simulink model "BalanceCar"  (R2022a)
settings: Solver=FixedStepDiscrete  StartTime=0.0  StopTime=inf  FixedStep=0.001  MaxStep=1e-3  RelTol=1e-3
values from neighbouring files (symbols this model uses):
  BALANCE_KD = 0.09    [BalanceCar.sldd]
  BALANCE_KP = 40.0    [BalanceCar.sldd]
  DIRECTION_KD = 0.1    [BalanceCar.sldd]
  DIRECTION_KP = 10.0    [BalanceCar.sldd]
  HIGH = 1.0    [BalanceCar.sldd]
  LOW = 0.0    [BalanceCar.sldd]
  MAX_PWM = 999.0    [BalanceCar.sldd]
  MIN_PWM = 900.0    [BalanceCar.sldd]
  NUM0 = 0.0    [BalanceCar.sldd]
  SPEED_KD = 0.0    [BalanceCar.sldd]
  SPEED_KI = 0.01    [BalanceCar.sldd]
  SPEED_KP = 18.0    [BalanceCar.sldd]
libraries: slpidlib x1
settings Model: DataDictionary=BalanceCar.sldd  Creator=Jepson  LastModifiedBy=Jepson
settings OptimizationCC: StrengthReduction=on  PassReuseOutputArgsAs=Individual arguments  ZeroExternalMemoryAtStartup=off  ZeroInternalMemoryAtStartup=off  NoFixptDivByZeroProtection=on  EfficientFloat2IntCast=on  OptimizeBlockOrder=speed  OptimizationPriority=Speed  MultiThreadedLoops=on  EfficientTunableParamExpr=on
settings DebuggingCC: ParameterPrecisionLossMsg=none  ParameterTunabilityLossMsg=error
settings HardwareCC: ProdBitPerPointer=32  ProdBitPerSizeT=32  ProdBitPerPtrDiffT=32  ProdLargestAtomicFloat=None  ProdWordSize=32  ProdHWDeviceType=Custom Processor->Custom Processor  TargetIntDivRoundTo=Zero  TargetEndianess=LittleEndian  TargetHWDeviceType=Custom Processor->Custom Processor  ProdEqTarget=off
settings ModelReferenceCC: ModelReferenceNumInstancesAllowed=Single
settings SFSimCC: MATLABDynamicMemAlloc=off
settings RTWCC: SystemTargetFile=ert.tlc  GenCodeOnly=on  TemplateMakefile=ert_default_tmf
settings CodeAppCC: ForceParamTrailComments=on  IgnoreCustomStorageClasses=off  OperatorAnnotations=on  SimulinkDataObjDesc=on  SFDataObjDesc=on  InsertBlockDesc=on
settings ERTTargetCC: TargetLangStandard=C99 (ISO)  GenerateSampleERTMain=on  IncludeMdlTerminateFcn=off  SupportNonFinite=off  SupportComplex=off  RemoveDisableFunc=on  ERTCustomFileTemplate=example_file_process.tlc  ERTFilePackagingFormat=CompactWithDataFile

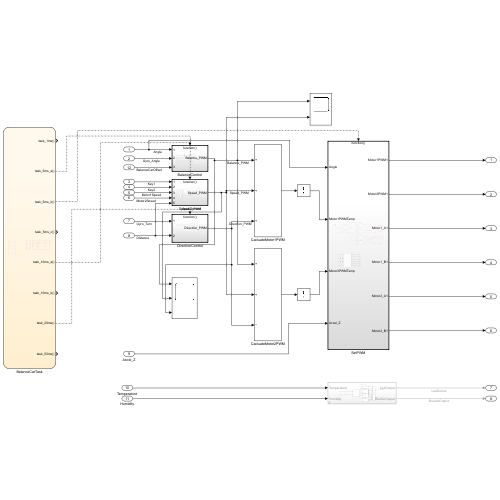
[thumbnail: Simulink's stored preview of the top-level diagram]
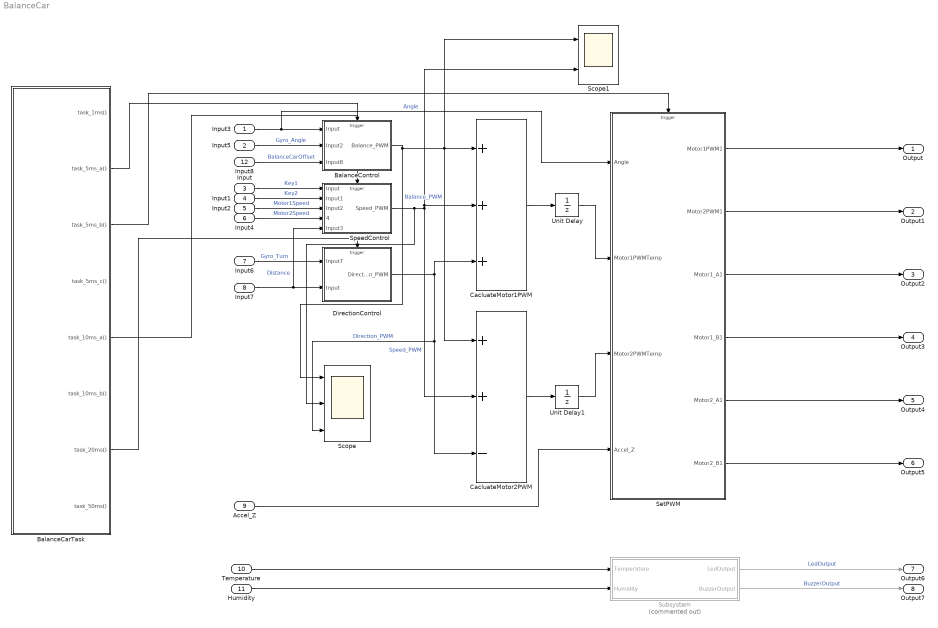
== system BalanceCar ==
  Input3 : Inport
  Input5 : Inport  Port=2
  Input : Inport  Port=3
  Input1 : Inport  Port=4
  Input2 : Inport  Port=5
  Input4 : Inport  Port=6
  Input6 : Inport  Port=7
  Input7 : Inport  Port=8
  Accel_Z : Inport  Port=9
  Temperature : Inport  Port=10
  Humidity : Inport  Port=11
  Input8 : Inport  Port=12
  BalanceCarTask : Stateflow chart  TreatAsAtomicUnit=on
      settings: PortSchema="{\"entries\":[{\"content\":{\"sides\":[{\"content\":{\"connectorIds\":[]},\"type\":\"ConnectorPlacement.EquallySpacedRectSide\",\"uuid\":\"98753e40-222e-4eaa-8b46-951d80aed91d\"},{\"content\":{\"connectorIds\":[\"Out2\",\"Out3\",\"Out5\",\"Out6\",\"Out1\",\"Out7\",\"Out4\",\"Out8\"],\"side\":\"RIGHT\"},\"type\":\"ConnectorPlacement.EquallySpacedRectSide\",\"uuid\":\"89dfa4e3-f29a-46ce-86e2-d4de18f5cc28\"},{\"content\":{\"connectorIds\":[],\"side\":\"TOP\"},\"type\":\"ConnectorPlacement.EquallySpacedRectSide\",\"uuid\":\"b5891d09-d472-4237-aaa4-93c027884cfd\"}]},\"type\":\"ConnectorPlacement.EquallySpacedConnector\",\"uuid\":\"b61f173b-e366-4c49-aaca-29ddc1ea1eb2\"}],\"packageUris\":[\"http://schema.mathworks.com/mf0/Connector/R2020b\"],\"version\":\"1.0\"}"
  BalanceControl : Subsystem  TreatAsAtomicUnit=on
      settings: RTWFcnNameOpts=Use subsystem name
  CacluateMotor1PWM : Sum  Inputs=+++
  CacluateMotor2PWM : Sum  Inputs=++-
  DirectionControl : Subsystem  TreatAsAtomicUnit=on  RTWFcnName=DirectionControl
      settings: RTWSystemCode=Nonreusable function  RTWFcnNameOpts=User specified
  Scope : Scope  NumInputPorts=3
  Scope1 : Scope  NumInputPorts=2
  SetPWM : Subsystem  TreatAsAtomicUnit=on
      settings: RTWFcnNameOpts=Use subsystem name
  SpeedControl : Subsystem  TreatAsAtomicUnit=on  RTWFcnName=SpeedControl
      settings: RTWSystemCode=Nonreusable function  RTWFcnNameOpts=User specified
  Subsystem : Subsystem  Commented=on
  Unit Delay : UnitDelay  SampleTime=-1  HasFrameUpgradeWarning=on
  Unit Delay1 : UnitDelay  SampleTime=-1  HasFrameUpgradeWarning=on
  Output : Outport
  Output1 : Outport  Port=2
  Output2 : Outport  Port=3
  Output3 : Outport  Port=4
  Output4 : Outport  Port=5
  Output5 : Outport  Port=6
  Output6 : Outport  Port=7
  Output7 : Outport  Port=8
  wires:
  Input/1 -> SpeedControl/1(Input)  "Key1"
  Input1/1 -> SpeedControl/2(Input1)  "Key2"
  Input2/1 -> SpeedControl/3(Input2)  "Motor1Speed"
  BalanceCarTask/3(task_5ms_a()) -> BalanceControl/Trigger
  Input3/1 -> BalanceControl/1(Input), SetPWM/1(Angle)  "Angle"
  Input5/1 -> BalanceControl/2(Input2)  "Gyro_Angle"
  BalanceControl/1(Balance_PWM) -> Scope1/1, CacluateMotor2PWM/1, CacluateMotor1PWM/1, Scope/1  "Balance_PWM"
  SpeedControl/1(Speed_PWM) -> Scope/2, Scope1/2, CacluateMotor1PWM/2, CacluateMotor2PWM/2  "Speed_PWM"
  SetPWM/1(Motor1PWM1) -> Output/1
  SetPWM/2(Motor2PWM1) -> Output1/1
  SetPWM/3(Motor1_A1) -> Output2/1
  SetPWM/4(Motor1_B1) -> Output3/1
  SetPWM/5(Motor2_A1) -> Output4/1
  SetPWM/6(Motor2_B1) -> Output5/1
  CacluateMotor1PWM/1 -> Unit Delay/1
  CacluateMotor2PWM/1 -> Unit Delay1/1
  Unit Delay/1 -> SetPWM/2(Motor1PWMTemp)
  Unit Delay1/1 -> SetPWM/3(Motor2PWMTemp)
  Input4/1 -> SpeedControl/4(4)  "Motor2Speed"
  BalanceCarTask/5(task_5ms_b()) -> SetPWM/Trigger
  BalanceCarTask/1(task_10ms_a()) -> SpeedControl/Trigger
  BalanceCarTask/4(task_20ms()) -> DirectionControl/Trigger
  Input7/1 -> SpeedControl/5(Input3), DirectionControl/2(Input)  "Distance"
  Input6/1 -> DirectionControl/1(Input7)  "Gyro_Turn"
  DirectionControl/1(Direction_PWM) -> CacluateMotor1PWM/3, CacluateMotor2PWM/3, Scope/3  "Direction_PWM"
  Accel_Z/1 -> SetPWM/4(Accel_Z)
  Temperature/1 -> Subsystem/1(Temperature)
  Humidity/1 -> Subsystem/2(Humidity)
  Subsystem/1(LedOutput) -> Output6/1  "LedOutput"
  Subsystem/2(BuzzerOutput) -> Output7/1  "BuzzerOutput"
  Input8/1 -> BalanceControl/3(Input8)  "BalanceCarOffset"

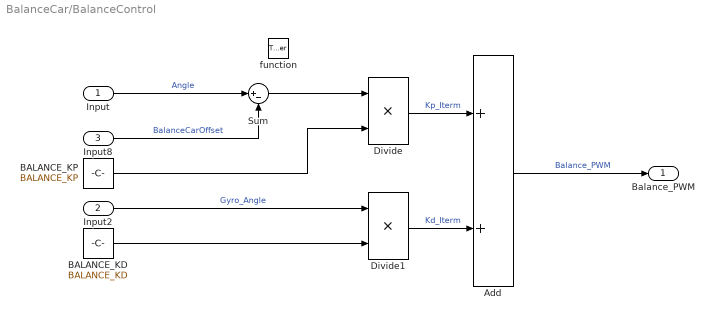
== system BalanceCar/BalanceControl ==
  Input : Inport
  Input2 : Inport  Port=2
  Input8 : Inport  Port=3
  function : TriggerPort  TriggerType=function-call  VariantControl=(inherit)
  Add : Sum  OutDataTypeStr=int16
  BALANCE_KD : Constant  Value=BALANCE_KD
  BALANCE_KP : Constant  Value=BALANCE_KP
  Divide : Product  Inputs=**
  Divide1 : Product  Inputs=**
  Sum : Sum  Inputs=|+-
  Balance_PWM : Outport
  wires:
  Input/1 -> Sum/1  "Angle"
  Sum/1 -> Divide/1
  Divide/1 -> Add/1  "Kp_Iterm"
  Input2/1 -> Divide1/1  "Gyro_Angle"
  Divide1/1 -> Add/2  "Kd_Iterm"
  Add/1 -> Balance_PWM/1  "Balance_PWM"
  Input8/1 -> Sum/2  "BalanceCarOffset"
  BALANCE_KP/1 -> Divide/2
  BALANCE_KD/1 -> Divide1/2

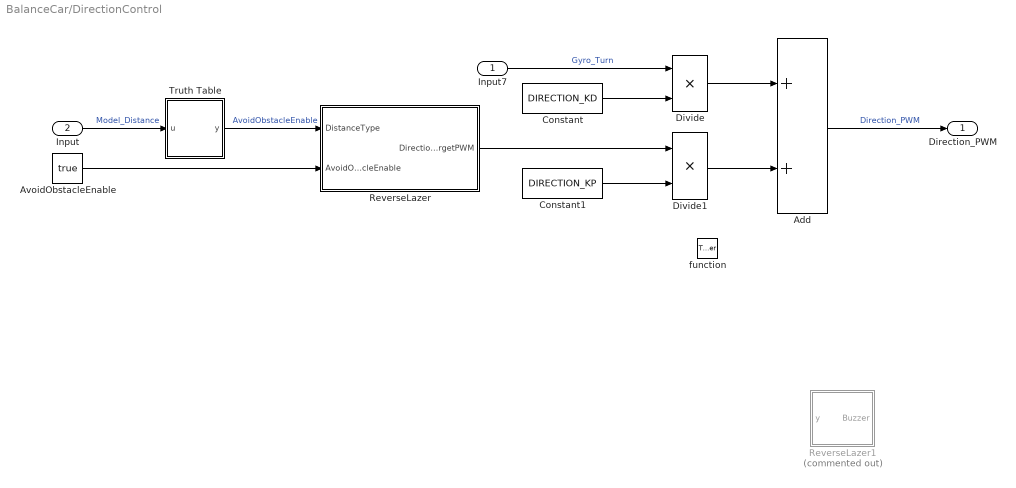
== system BalanceCar/DirectionControl ==
  Input7 : Inport
  Input : Inport  Port=2
  function : TriggerPort  TriggerType=function-call  VariantControl=(inherit)
  Add : Sum  OutDataTypeStr=int16
  AvoidObstacleEnable : Constant  Value=true  OutDataTypeStr=boolean
  Constant : Constant  Value=DIRECTION_KD
  Constant1 : Constant  Value=DIRECTION_KP
  Divide : Product  Inputs=**
  Divide1 : Product  Inputs=**
  ReverseLazer : Stateflow chart  TreatAsAtomicUnit=on
  ReverseLazer1 : Stateflow chart  Commented=on  TreatAsAtomicUnit=on
  Truth Table : Truth Table  TreatAsAtomicUnit=on
      settings: RTWSystemCode=Nonreusable function
  Direction_PWM : Outport
  wires:
  Input/1 -> Truth Table/1(u)  "Model_Distance"
  Truth Table/1(y) -> ReverseLazer/1(DistanceType)  "AvoidObstacleEnable"
  Input7/1 -> Divide/1  "Gyro_Turn"
  Constant/1 -> Divide/2
  Constant1/1 -> Divide1/2
  Divide/1 -> Add/1
  Divide1/1 -> Add/2
  Add/1 -> Direction_PWM/1  "Direction_PWM"
  ReverseLazer/1(DirectionTargetPWM) -> Divide1/1
  AvoidObstacleEnable/1 -> ReverseLazer/2(AvoidObstacleEnable)

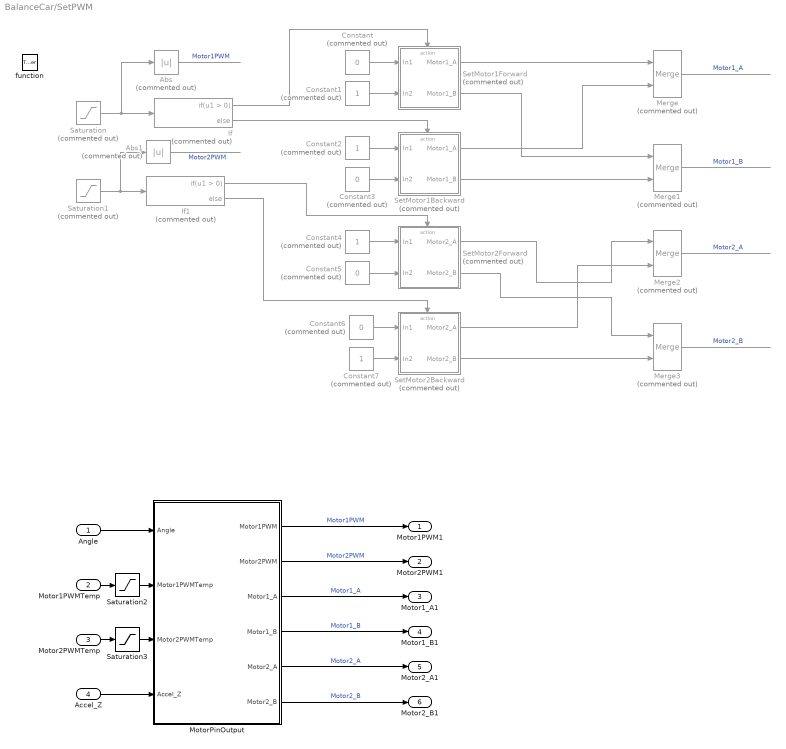
== system BalanceCar/SetPWM ==
  Angle : Inport
  Motor1PWMTemp : Inport  Port=2
  Motor2PWMTemp : Inport  Port=3
  Accel_Z : Inport  Port=4
  function : TriggerPort  TriggerType=function-call  VariantControl=(inherit)
  Abs : Abs  Commented=on  OutDataTypeStr=uint16  SaturateOnIntegerOverflow=off
  Abs1 : Abs  Commented=on  OutDataTypeStr=uint16  SaturateOnIntegerOverflow=off
  Constant{,3,5..6} (4 alike) : Constant  Commented=on  Value=0  OutDataTypeStr=uint8
  Constant{1..2,4,7} (4 alike) : Constant  Commented=on  OutDataTypeStr=uint8
  If : If  Commented=on
  If1 : If  Commented=on
  Merge{,1..3} (4 alike) : Merge  Commented=on
  MotorPinOutput : Stateflow chart  TreatAsAtomicUnit=on
      settings: PortSchema="{\"entries\":[{\"content\":{\"sides\":[{\"content\":{\"connectorIds\":[\"In3\",\"In1\",\"In2\",\"In4\"]},\"type\":\"ConnectorPlacement.EquallySpacedRectSide\",\"uuid\":\"f3e6de76-1fe1-4774-9311-d7aaff92af40\"},{\"content\":{\"connectorIds\":[\"Out1\",\"Out2\",\"Out3\",\"Out4\",\"Out5\",\"Out6\"],\"side\":\"RIGHT\"},\"type\":\"ConnectorPlacement.EquallySpacedRectSide\",\"uuid\":\"9ddd8262-d02c-4418-a44c-aa5250dd09ec\"},{\"content\":{\"connectorIds\":[],\"side\":\"TOP\"},\"type\":\"ConnectorPlacement.EquallySpacedRectSide\",\"uuid\":\"74ca197d-86c3-441f-a010-8590a39af9cb\"}]},\"type\":\"ConnectorPlacement.EquallySpacedConnector\",\"uuid\":\"3610e4e7-604b-4874-a455-67045648e8e5\"}],\"packageUris\":[\"http://schema.mathworks.com/mf0/Connector/R2020b\"],\"version\":\"1.0\"}"
  Saturation : Saturate  Commented=on  UpperLimit=900  LowerLimit=-900  OutDataTypeStr=int16
  Saturation1 : Saturate  Commented=on  UpperLimit=900  LowerLimit=-900  OutDataTypeStr=int16
  Saturation2 : Saturate  UpperLimit=990  LowerLimit=-900
  Saturation3 : Saturate  UpperLimit=999  LowerLimit=-999
  SetMotor1Backward : Subsystem  Commented=on  TreatAsAtomicUnit=on
  SetMotor1Forward : Subsystem  Commented=on  TreatAsAtomicUnit=on
  SetMotor2Backward : Subsystem  Commented=on  TreatAsAtomicUnit=on
  SetMotor2Forward : Subsystem  Commented=on  TreatAsAtomicUnit=on
  Motor1PWM1 : Outport
  Motor2PWM1 : Outport  Port=2
  Motor1_A1 : Outport  Port=3
  Motor1_B1 : Outport  Port=4
  Motor2_A1 : Outport  Port=5
  Motor2_B1 : Outport  Port=6
  wires:
  If/1 -> SetMotor1Forward/Action
  Constant/1 -> SetMotor1Forward/1(In1)
  Constant1/1 -> SetMotor1Forward/2(In2)
  If/2 -> SetMotor1Backward/Action
  Constant3/1 -> SetMotor1Backward/2(In2)
  Constant2/1 -> SetMotor1Backward/1(In1)
  Abs/1 -> ?  "Motor1PWM"
  Abs1/1 -> ?  "Motor2PWM"
  Constant6/1 -> SetMotor2Backward/1(In1)
  Constant7/1 -> SetMotor2Backward/2(In2)
  If1/2 -> SetMotor2Backward/Action
  Constant5/1 -> SetMotor2Forward/2(In2)
  Constant4/1 -> SetMotor2Forward/1(In1)
  If1/1 -> SetMotor2Forward/Action
  SetMotor1Forward/1(Motor1_A) -> Merge/1
  SetMotor1Backward/1(Motor1_A) -> Merge/2
  Merge/1 -> ?  "Motor1_A"
  SetMotor1Backward/2(Motor1_B) -> Merge1/2
  SetMotor1Forward/2(Motor1_B) -> Merge1/1
  SetMotor2Forward/1(Motor2_A) -> Merge2/1
  SetMotor2Backward/1(Motor2_A) -> Merge2/2
  SetMotor2Forward/2(Motor2_B) -> Merge3/1
  SetMotor2Backward/2(Motor2_B) -> Merge3/2
  Merge1/1 -> ?  "Motor1_B"
  Merge2/1 -> ?  "Motor2_A"
  Merge3/1 -> ?  "Motor2_B"
  MotorPinOutput/5(Motor2_A) -> Motor2_A1/1  "Motor2_A"
  MotorPinOutput/6(Motor2_B) -> Motor2_B1/1  "Motor2_B"
  MotorPinOutput/2(Motor2PWM) -> Motor2PWM1/1  "Motor2PWM"
  MotorPinOutput/1(Motor1PWM) -> Motor1PWM1/1  "Motor1PWM"
  MotorPinOutput/4(Motor1_B) -> Motor1_B1/1  "Motor1_B"
  MotorPinOutput/3(Motor1_A) -> Motor1_A1/1  "Motor1_A"
  Saturation1/1 -> Abs1/1, If1/1
  Saturation/1 -> Abs/1, If/1
  Angle/1 -> MotorPinOutput/3(Angle)
  Motor1PWMTemp/1 -> Saturation2/1
  Motor2PWMTemp/1 -> Saturation3/1
  Saturation2/1 -> MotorPinOutput/1(Motor1PWMTemp)
  Saturation3/1 -> MotorPinOutput/2(Motor2PWMTemp)
  Accel_Z/1 -> MotorPinOutput/4(Accel_Z)

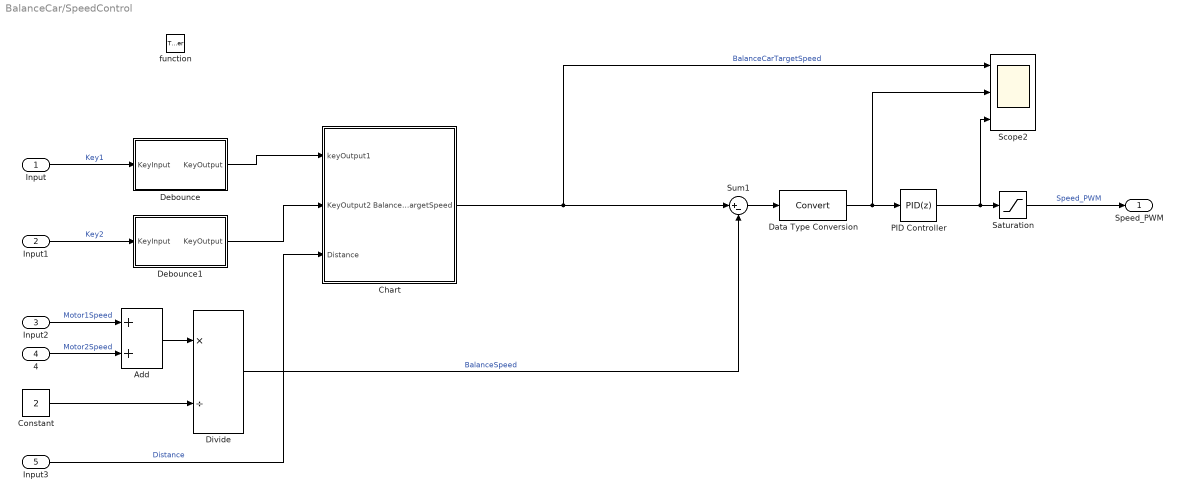
== system BalanceCar/SpeedControl ==
  Input : Inport
  Input1 : Inport  Port=2
  Input2 : Inport  Port=3
  4 : Inport  Port=4
  Input3 : Inport  Port=5
  function : TriggerPort  TriggerType=function-call  VariantControl=(inherit)
  Add : Sum
  Chart : Stateflow chart  TreatAsAtomicUnit=on
  Constant : Constant  Value=2  OutDataTypeStr=int8
  Data Type Conversion : DataTypeConversion  SaturateOnIntegerOverflow=off  RndMeth=Floor
  Debounce : Stateflow chart  TreatAsAtomicUnit=on
  Debounce1 : Stateflow chart  TreatAsAtomicUnit=on
  Divide : Product  Inputs=*/  OutDataTypeStr=int16
  PID Controller : slpidlib/PID Controller  Controller=PID  Form=Parallel  TimeDomain=Discrete-time  UseExternalTs=off  SampleTime=-1  IntegratorMethod=Forward Euler  FilterMethod=Forward Euler  ControllerParametersSource=internal  P=SPEED_KP  I=SPEED_KI  UseKiTs=on  D=SPEED_KD  N=100  UseFilter=on  TunerSelectOption=Transfer Function Based (PID Tuner App)  InitialConditionSource=internal  InitialConditionForIntegrator=0  InitialConditionForFilter=0  DifferentiatorICPrevScaledInput=0  ExternalReset=none  TrackingMode=off  Kt=1  LimitOutput=off  SatLimitsSource=internal  UpperSaturationLimit=MAX_PWM  LowerSaturationLimit=MIN_PWM  LinearizeAsGain=off  AntiWindupMode=none  Kb=1  POutMin=[]  POutMax=[]  IOutMin=[]  IOutMax=[]  DOutMin=[]  DOutMax=[]  NOutMin=[]  NOutMax=[]  SumOutDataTypeStr=int16  SumOutMin=[]  SumOutMax=[]  SaturationOutMin=[]  SaturationOutMax=[]  PParamMin=[]  PParamMax=[]  IParamMin=[]  IParamMax=[]  DParamMin=[]  DParamMax=[]  NParamMin=[]  NParamMax=[]  KbParamMin=[]  KbParamMax=[]  KtParamMin=[]  KtParamMax=[]  KbOutMin=[]  KbOutMax=[]  KtOutMin=[]  KtOutMax=[]  IntegratorOutMin=[]  IntegratorOutMax=[]  FilterOutMin=[]  FilterOutMax=[]  SumI1OutMin=[]  SumI1OutMax=[]  SumI2OutMin=[]  SumI2OutMax=[]  SumI3OutMin=[]  SumI3OutMax=[]  SumI4OutMin=[]  SumI4OutMax=[]  SumDOutMin=[]  SumDOutMax=[]  DifferentiatorOutMin=[]  DifferentiatorOutMax=[]  FilterDiffOutCoefMin=[]  FilterDiffOutCoefMax=[]  ReciprocalOutMin=[]  ReciprocalOutMax=[]  SumDenOutMin=[]  SumDenOutMax=[]  SumNumOutMin=[]  SumNumOutMax=[]  DivideOutMin=[]  DivideOutMax=[]  UdiffTsProdOutMin=[]  UdiffTsProdOutMax=[]  NTsProdOutMin=[]  NTsProdOutMax=[]  UintegralTsProdOutMin=[]  UintegralTsProdOutMax=[]  UngainTsProdOutMin=[]  UngainTsProdOutMax=[]  ClampingZeroOutDataTypeStr=Inherit: Inherit via back propagation  ClampingZeroOutMin=[]  ClampingZeroOutMax=[]  FilterDenConstantOutDataTypeStr=Inherit: Inherit via back propagation  FilterDenConstantOutMin=[]  FilterDenConstantOutMax=[]  PCopyOutDataTypeStr=Inherit: Inherit via back propagation  PCopyOutMin=[]  PCopyOutMax=[]  NCopyOutDataTypeStr=Inherit: Inherit via back propagation  NCopyOutMin=[]  NCopyOutMax=[]  IntegratorContinuousStateAttributes=''  IntegratorStateMustResolveToSignalObject=off  IntegratorRTWStateStorageClass=Auto  FilterContinuousStateAttributes=''  FilterStateMustResolveToSignalObject=off  FilterRTWStateStorageClass=Auto  ParallelPVariant=InternalParameters  IdealPVariant=Disabled  IVariant=InternalParameters  DVariant=InternalParameters  IntegratorVariant=Discrete  SatVariant=Disabled  AWVariant=Passthrough  PCopyVariant=Disabled  TRVariant=Disabled  FdbkBlocksVariant=Forward  IdealPFdbkVariant=Disabled  SatFdbkVariant=Disabled  DerivativeFilterVariant=ForwardEulerFilter  NVariant=InternalParameters  NCopyVariant=Disabled  FilterICVariant=InternalICsFilter  IntegratorICVariant=InternalICs  ExternalResetVariant=Disabled  TRSumVariant=Passthrough  SumFdbkVariant=Disabled  SumVariant=Sum_PID  TsampFilterVariant=InternalTs  TsampNgainVariant=Passthrough  TsampIntegralVariant=Passthrough  ExternalSaturationOutDataTypeStr=Inherit: Same as second input  aMode=0
  Saturation : Saturate  UpperLimit=900  LowerLimit=-900  OutDataTypeStr=int16
  Scope2 : Scope  NumInputPorts=3
  Sum1 : Sum  Inputs=|+-  InputSameDT=on  OutDataTypeStr=int16  LockScale=on
  Speed_PWM : Outport  OutDataTypeStr=int16
  wires:
  Input/1 -> Debounce/1(KeyInput)  "Key1"
  Debounce/1(KeyOutput) -> Chart/1(keyOutput1)
  Chart/1(BalanceCarTargetSpeed) -> Scope2/1, Sum1/1  "BalanceCarTargetSpeed"
  Debounce1/1(KeyOutput) -> Chart/2(KeyOutput2)
  Input1/1 -> Debounce1/1(KeyInput)  "Key2"
  Data Type Conversion/1 -> Scope2/2, PID Controller/1
  Sum1/1 -> Data Type Conversion/1
  PID Controller/1 -> Saturation/1, Scope2/3
  Input2/1 -> Add/1  "Motor1Speed"
  4/1 -> Add/2  "Motor2Speed"
  Add/1 -> Divide/1
  Constant/1 -> Divide/2
  Divide/1 -> Sum1/2  "BalanceSpeed"
  Saturation/1 -> Speed_PWM/1  "Speed_PWM"
  Input3/1 -> Chart/3(Distance)  "Distance"

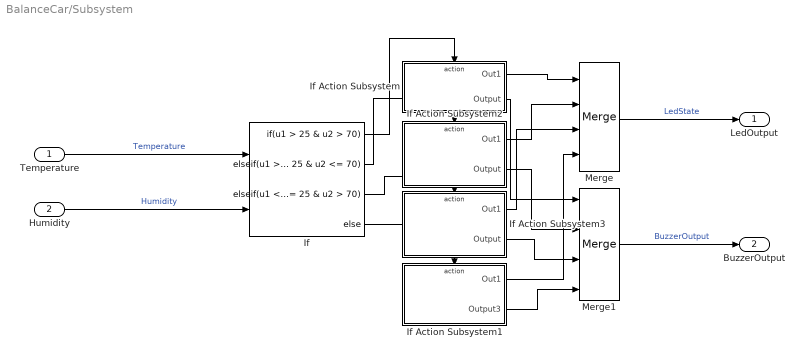
== system BalanceCar/Subsystem ==
  Temperature : Inport
  Humidity : Inport  Port=2
  If : If  NumInputs=2  IfExpression=u1 > 25 & u2 > 70  ElseIfExpressions=u1 > 25 & u2 <= 70,u1 <= 25 & u2 > 70
  If Action Subsystem : Subsystem  TreatAsAtomicUnit=on
  If Action Subsystem1 : Subsystem  TreatAsAtomicUnit=on
  If Action Subsystem2 : Subsystem  TreatAsAtomicUnit=on
  If Action Subsystem3 : Subsystem  TreatAsAtomicUnit=on
  Merge : Merge  Inputs=4
  Merge1 : Merge  Inputs=4
  LedOutput : Outport
  BuzzerOutput : Outport  Port=2
  wires:
  If/2 -> If Action Subsystem2/Action
  If/1 -> If Action Subsystem/Action
  If/4 -> If Action Subsystem1/Action
  If Action Subsystem1/2(Output3) -> Merge1/4
  If Action Subsystem3/2(Output) -> Merge1/3
  If Action Subsystem2/1(Out1) -> Merge/2
  If Action Subsystem2/2(Output) -> Merge1/2
  If Action Subsystem3/1(Out1) -> Merge/3
  If/3 -> If Action Subsystem3/Action
  If Action Subsystem1/1(Out1) -> Merge/4
  If Action Subsystem/2(Output) -> Merge1/1
  If Action Subsystem/1(Out1) -> Merge/1
  Temperature/1 -> If/1  "Temperature"
  Merge/1 -> LedOutput/1  "LedState"
  Merge1/1 -> BuzzerOutput/1  "BuzzerOutput"
  Humidity/1 -> If/2  "Humidity"

== system BalanceCar/SetPWM/MotorPinOutput/abs ==
  x : Inport  OutDataTypeStr=int16  PortDimensions=1
  f : TriggerPort  TriggerType=function-call  VariantControl=(inherit)
      settings: CopyFcn=Stateflow.SLINSF.SimulinkMan.removeBlockPreDeleteFcn  PreDeleteFcn=Stateflow.SLINSF.SimulinkMan.unsafePredeleteFcn
  Abs : Abs  OutDataTypeStr=uint16  SaturateOnIntegerOverflow=off
  y : Outport  OutDataTypeStr=uint16
  wires:
  x/1 -> Abs/1
  Abs/1 -> y/1

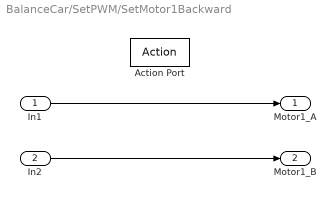
== system BalanceCar/SetPWM/SetMotor1Backward ==
  In1 : Inport
  In2 : Inport  Port=2
  Action Port : ActionPort  ActionPortLabel=else
  Motor1_A : Outport
  Motor1_B : Outport  Port=2
  wires:
  In2/1 -> Motor1_B/1
  In1/1 -> Motor1_A/1

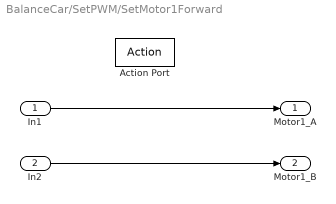
== system BalanceCar/SetPWM/SetMotor1Forward ==
  In1 : Inport
  In2 : Inport  Port=2
  Action Port : ActionPort  ActionPortLabel=if(u1 > 0)
  Motor1_A : Outport
  Motor1_B : Outport  Port=2
  wires:
  In2/1 -> Motor1_B/1
  In1/1 -> Motor1_A/1

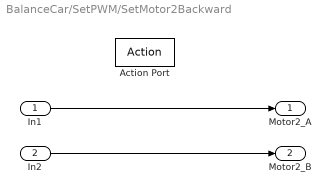
== system BalanceCar/SetPWM/SetMotor2Backward ==
  In1 : Inport
  In2 : Inport  Port=2
  Action Port : ActionPort  ActionPortLabel=else
  Motor2_A : Outport
  Motor2_B : Outport  Port=2
  wires:
  In1/1 -> Motor2_A/1
  In2/1 -> Motor2_B/1

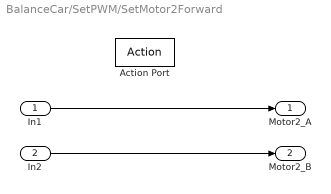
== system BalanceCar/SetPWM/SetMotor2Forward ==
  In1 : Inport
  In2 : Inport  Port=2
  Action Port : ActionPort  ActionPortLabel=if(u1 > 0)
  Motor2_A : Outport
  Motor2_B : Outport  Port=2
  wires:
  In1/1 -> Motor2_A/1
  In2/1 -> Motor2_B/1

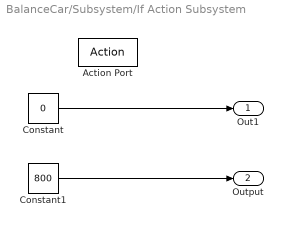
== system BalanceCar/Subsystem/If Action Subsystem ==
  Action Port : ActionPort  ActionPortLabel=if(u1 > 25 & u2 > 70)
  Constant : Constant  Value=0  OutDataTypeStr=uint8
  Constant1 : Constant  Value=800  OutDataTypeStr=uint16
  Out1 : Outport
  Output : Outport  Port=2
  wires:
  Constant/1 -> Out1/1
  Constant1/1 -> Output/1

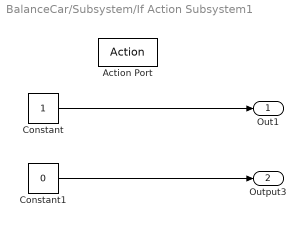
== system BalanceCar/Subsystem/If Action Subsystem1 ==
  Action Port : ActionPort  ActionPortLabel=else
  Constant : Constant  OutDataTypeStr=uint8
  Constant1 : Constant  Value=0  OutDataTypeStr=uint16
  Out1 : Outport
  Output3 : Outport  Port=2
  wires:
  Constant/1 -> Out1/1
  Constant1/1 -> Output3/1

== system BalanceCar/Subsystem/If Action Subsystem2 ==
  Action Port : ActionPort  ActionPortLabel=elseif(u1 > 25 & u2 <= 70)
  Constant : Constant  Value=0  OutDataTypeStr=uint8
  Constant1 : Constant  Value=0  OutDataTypeStr=uint16
  Out1 : Outport
  Output : Outport  Port=2
  wires:
  Constant1/1 -> Output/1
  Constant/1 -> Out1/1

== system BalanceCar/Subsystem/If Action Subsystem3 ==
  Action Port : ActionPort  ActionPortLabel=elseif(u1 <= 25 & u2 > 70)
  Constant : Constant  OutDataTypeStr=uint8
  Constant1 : Constant  Value=800  OutDataTypeStr=uint16
  Out1 : Outport
  Output : Outport  Port=2
  wires:
  Constant/1 -> Out1/1
  Constant1/1 -> Output/1

== stateflow chart BalanceCar/DirectionControl/ReverseLazer ==
  state Default [commented out]
    en:
    DirectionTargetPWM = 0;
    du:
    % disable chaoshengbo
    DiasbleAvoidObstacle = false;
  state TurnDirection [commented out]
    en:
    DirectionTargetPWM = 20;
    du:
    DirectionTargetPWM = DirectionTargetPWM - 1;
  state Back [commented out]
    en:
    DirectionTargetPWM = -20;
    du:
    DirectionTargetPWM = DirectionTargetPWM + 1;
  state Default1
    en:
    DirectionTargetPWM = 0;
  state TurnDirection1
    en:
    DirectionTargetPWM = 0;
    state Enter1
      du:
      DirectionTargetPWM = DirectionTargetPWM + 5;
    state End1
    (default) -> TurnDirection1.Enter1
    TurnDirection1.Enter1 -> TurnDirection1.End1 : [ DistanceType == 0 || DirectionTargetPWM > 100]
  state StopTurn
    en:
    state Enter1
      du:
      DirectionTargetPWM = DirectionTargetPWM - 10;
    state End1
    (default) -> StopTurn.Enter1
    StopTurn.Enter1 -> StopTurn.End1 : [DirectionTargetPWM == 0]
  state Back2 [commented out]
    en:
    DirectionTargetPWM = 40;
    state Enter1 [commented out]
      du:
      DirectionTargetPWM = DirectionTargetPWM - 4;
    state End1 [commented out]
    (default) -> Back2.Enter1 [commented out]
    Back2.Enter1 -> Back2.End1 [commented out] : [DirectionTargetPWM == 0]
  state Back1 [commented out]
    en:
    DirectionTargetPWM = 40;
    state Enter1 [commented out]
      du:
      DirectionTargetPWM = DirectionTargetPWM - 4;
    state End1 [commented out]
    (default) -> Back1.Enter1 [commented out]
    Back1.Enter1 -> Back1.End1 [commented out] : [DirectionTargetPWM == 0]
  (default) -> Default [commented out]
  Default -> TurnDirection [commented out] : [DiasbleAvoidObstacle...
      | &&(DistanceType == 1 || DistanceType == 2 || DistanceType == 3)]
  TurnDirection -> Back [commented out] : [(DirectionTargetPWM == 0)&&after(1000,msec)]
  Back -> Default [commented out] : [(DirectionTargetPWM == 0)&&after(1000,msec)]
  (default) -> Default1
  Default1 -> TurnDirection1 : [AvoidObstacleEnable...
      |  &&(DistanceType == 1)...
      |  &&(DistanceType == 2)...
      |  &&(DistanceType == 3)]
  TurnDirection1.End1 -> StopTurn : [after(10,msec)]
  StopTurn -> Default1 : [DirectionTargetPWM == 0 || DistanceType == 0]
  StopTurn.End1 -> Back2 [commented out] : [after(20,msec)]
  Back2.End1 -> Back1 [commented out] : [after(20,msec)]
  data: DirectionTargetPWM output; DistanceType input; AvoidObstacleEnable input

== matlab function BalanceCar/DirectionControl/Truth Table ==
  data: u input; y output uint8 =0
function y = fcn(u)

aVarTruthTableCondition_1 = false;
aVarTruthTableCondition_2 = false;
aVarTruthTableCondition_3 = false;


% Example condition 1

aVarTruthTableCondition_1 = logical((u  <= 10) &&(u  >=0));

% Example condition 2

aVarTruthTableCondition_2 = logical((u  <= 30) &&(u  > 10));

% Example condition 3

aVarTruthTableCondition_3 = logical((u  >30) &&(u  < 50));

if (aVarTruthTableCondition_1)
    aFcnTruthTableAction_1();
elseif (~aVarTruthTableCondition_1 && aVarTruthTableCondition_2)
    aFcnTruthTableAction_2();
elseif (~aVarTruthTableCondition_1 && ~aVarTruthTableCondition_2 && aVarTruthTableCondition_3)
    aFcnTruthTableAction_3();
else % Default
    aFcnTruthTableAction_4();
end

function aFcnTruthTableAction_1()

% Action 1:Dangerous

y = 1;

function aFcnTruthTableAction_2()

% Action 2: Carefull

y = 2;

function aFcnTruthTableAction_3()

% Action 3:Warning

y = 3;

function aFcnTruthTableAction_4()

% Action 4:Noramal

y = 0;

== stateflow chart BalanceCar/BalanceCarTask ==
  state Task_5ms [function]
    (default) -> (junction 132)
    (junction 132) -> (junction 140) [order 1] : [task_5ms_count == 1]
    (junction 132) -> (junction 144) [order 2]
    (junction 140) -> (junction 142) : {task_5ms_a}
    (junction 142) -> (junction 144)
    (junction 144) -> (junction 148)
    (junction 148) -> (junction 155) [order 1] : [task_5ms_count == 2]
    (junction 148) -> (junction 151) [order 2]
    (junction 155) -> (junction 152) : {task_5ms_b}
    (junction 152) -> (junction 151)
    (junction 151) -> (junction 162)
    (junction 162) -> (junction 166) [order 1] : [task_5ms_count == 3]
    (junction 162) -> (junction 160) [order 2]
    (junction 166) -> (junction 161) : {task_5ms_c}
    (junction 161) -> (junction 160)
  state Task_10ms [function]
    (default) -> (junction 169)
    (junction 169) -> (junction 193) [order 1] : [task_10ms_count == 2]
    (junction 169) -> (junction 181) [order 2]
    (junction 193) -> (junction 190) : {task_10ms_a}
    (junction 190) -> (junction 181)
    (junction 181) -> (junction 185)
    (junction 185) -> (junction 189) [order 1] : [task_10ms_count == 3]
    (junction 185) -> (junction 183) [order 2]
    (junction 189) -> (junction 184) : {task_10ms_b}
    (junction 184) -> (junction 183)
  state Task_20ms [function]
    (default) -> (junction 196)
    (junction 196) -> (junction 204) [order 1] : [task_20ms_count == 3]
    (junction 196) -> (junction 201) [order 2]
    (junction 204) -> (junction 202) : {task_20ms}
    (junction 202) -> (junction 201)
  state Task_50ms [function]
    (default) -> (junction 206)
    (junction 206) -> (junction 214) [order 1] : [task_50ms_count == 4]
    (junction 206) -> (junction 211) [order 2]
    (junction 214) -> (junction 212) : {task_50ms}
    (junction 212) -> (junction 211)
  (default) -> (junction 87) : {task_5ms_count = task_5ms_count + 1;}
  (junction 87) -> (junction 69) : {task_1ms;}
  (junction 69) -> (junction 77) [order 1] : [mod(task_5ms_count,5)==0]
  (junction 69) -> (junction 71) [order 2]
  (junction 77) -> (junction 79) : {task_5ms_count = 0;}
  (junction 79) -> (junction 71)
  (junction 71) -> (junction 93) : {task_10ms_count = task_10ms_count + 1;}
  (junction 93) -> (junction 95) [order 1] : [mod(task_10ms_count,10)==0]
  (junction 93) -> (junction 97) [order 2]
  (junction 95) -> (junction 99) : {task_10ms_count = 0;}
  (junction 99) -> (junction 97)
  (junction 97) -> (junction 106) : {task_20ms_count = task_20ms_count + 1;}
  (junction 106) -> (junction 108) [order 1] : [mod(task_20ms_count,20)==0]
  (junction 106) -> (junction 103) [order 2]
  (junction 108) -> (junction 109) : {task_20ms_count = 1;}
  (junction 109) -> (junction 103)
  (junction 103) -> (junction 114) : {task_50ms_count = task_50ms_count + 1;}
  (junction 114) -> (junction 117) [order 1] : [mod(task_50ms_count,50)==0]
  (junction 114) -> (junction 115) [order 2]
  (junction 117) -> (junction 116) : {task_50ms_count = 0;}
  (junction 116) -> (junction 115)
  (junction 115) -> (junction 138) : {Task_5ms();
      | Task_10ms();
      | Task_20ms();
      | Task_50ms();}
  data: task_5ms_count local uint8 =NUM0; task_10ms_count local uint8 =NUM0; task_20ms_count local uint8 =NUM0; task_50ms_count local uint8 =NUM0
  events: task_10ms_a output FUNCTION_CALL_EVENT; task_1ms output FUNCTION_CALL_EVENT; task_5ms_a output FUNCTION_CALL_EVENT; task_20ms output FUNCTION_CALL_EVENT; task_5ms_b output FUNCTION_CALL_EVENT; task_5ms_c output FUNCTION_CALL_EVENT; task_10ms_b output FUNCTION_CALL_EVENT; task_50ms output FUNCTION_CALL_EVENT

== stateflow chart BalanceCar/SpeedControl/Debounce ==
  state Debounce [parallel]
    settings: executionOrder=1
    state Key1Off
      du:
      KeyState = OFF;
    state KeyOn
      du:
      KeyState = ON;
      KeyOnFlag = true;
    (default) -> Key1Off
    Key1Off -> KeyOn : [duration(KeyInput <= NUM0)>=0.01]
    KeyOn -> Key1Off : [duration(KeyInput > NUM0)>=0.01]
  state KeyCounter [function]
    (default) -> (junction 40)
    (junction 40) -> (junction 43) [order 1] : [(KeyOnFlag == true)&&(KeyState == OFF)]
    (junction 40) -> (junction 41) [order 2]
    (junction 43) -> (junction 37) : {KeyOnFlag = false;
        | KeyOutput =  ON;}
    (junction 41) -> (junction 37) : {KeyOutput =  OFF;}
  state KeyTimes [parallel]
    du:
    KeyCounter();
    settings: executionOrder=2
  data: KeyInput input uint8; OFF parameter; ON parameter; NUM0 parameter; KeyOutput output uint8; KeyOnFlag local boolean =false; KeyState local uint8 =OFF

== stateflow chart BalanceCar/SpeedControl/Debounce1 ==
  state Debounce [parallel]
    settings: executionOrder=1
    state Key1Off
      du:
      KeyState = OFF;
    state KeyOn
      du:
      KeyState = ON;
      KeyOnFlag = true;
    (default) -> Key1Off
    Key1Off -> KeyOn : [duration(KeyInput <= NUM0)>=0.01]
    KeyOn -> Key1Off : [duration(KeyInput > NUM0)>=0.01]
  state KeyCounter [function]
    (default) -> (junction 40)
    (junction 40) -> (junction 43) [order 1] : [(KeyOnFlag == true)&&(KeyState == OFF)]
    (junction 40) -> (junction 41) [order 2]
    (junction 43) -> (junction 37) : {KeyOnFlag = false;
        | KeyOutput =  ON;}
    (junction 41) -> (junction 37) : {KeyOutput =  OFF;}
  state KeyTimes [parallel]
    du:
    KeyCounter();
    settings: executionOrder=2
  data: KeyInput input uint8; OFF parameter; ON parameter; NUM0 parameter; KeyOutput output uint8; KeyOnFlag local boolean =false; KeyState local uint8 =OFF

== stateflow chart BalanceCar/SpeedControl/Chart ==
  state SpeedDown [function]
    (default) -> (junction 33)
    (junction 33) -> (junction 35) [order 1] : [KeyOutput2 == ON]
    (junction 33) -> (junction 37) [order 2]
    (junction 35) -> (junction 41) : {BalanceCarTargetSpeed=BalanceCarTargetSpeed-20;}
    (junction 37) -> (junction 41)
  state SpeedUp [function]
    (default) -> (junction 26)
    (junction 26) -> (junction 28) [order 1] : [keyOutput1 == ON]
    (junction 26) -> (junction 30) [order 2]
    (junction 28) -> (junction 23) : {BalanceCarTargetSpeed=BalanceCarTargetSpeed+20;}
    (junction 30) -> (junction 23)
  state SpeedUpStatus
    en:
    BalanceCarTargetSpeed = 0;
    du:
    SpeedUp();
    SpeedDown();
    SpeedStop();
  state SpeedStop [function]
    (default) -> (junction 58)
    (junction 58) -> (junction 59) [order 1] : [Distance <= 10]
    (junction 58) -> (junction 60) [order 2]
    (junction 59) -> (junction 61)
    (junction 60) -> (junction 61)
  (default) -> SpeedUpStatus
  data: keyOutput1 input; ON parameter; KeyOutput2 input; BalanceCarTargetSpeed output int16; Distance input

== stateflow chart BalanceCar/DirectionControl/ReverseLazer1 ==
  state Dangours
    en:
    state RuningState
      du:
      Buzzer = 480;
    state StopState
      du:
      Buzzer = 0;
    (default) -> Dangours.RuningState
    Dangours.RuningState -> Dangours.StopState : [after(20,msec)]
    Dangours.StopState -> Dangours.RuningState : [after(10,msec)]
  state Default
    en:
    Buzzer = 0;
  state Warning
    state RuningState
      du:
      Buzzer = 480;
    state StopState
      du:
      Buzzer = 0;
    (default) -> Warning.RuningState
    Warning.RuningState -> Warning.StopState : [after(50,msec)]
    Warning.StopState -> Warning.RuningState : [after(20,msec)]
  state Careful
    state RuningState
      du:
      Buzzer = 480;
    state StopState
      du:
      Buzzer = 0;
    (default) -> Careful.RuningState
    Careful.RuningState -> Careful.StopState : [after(100,msec)]
    Careful.StopState -> Careful.RuningState : [after(50,msec)]
  state Normal
    en:
    Buzzer = 0;
  (default) -> Default
  Default -> Dangours [order 1] : [y == 1]
  Dangours -> Warning [order 1] : [y==2]
  Warning -> Dangours [order 1] : [y==1]
  Dangours -> Careful [order 3] : [y == 3]
  Careful -> Dangours [order 3] : [y==1]
  Normal -> Dangours [order 3] : [y==1]
  Dangours -> Normal [order 2] : [y==4]
  Default -> Warning [order 2] : [y==2]
  Warning -> Careful [order 2] : [y==3]
  Careful -> Warning [order 2] : [y==2]
  Warning -> Normal [order 3] : [y==4]
  Normal -> Warning [order 2] : [y==2]
  Default -> Careful [order 4] : [y == 3]
  Careful -> Normal [order 1] : [y==4]
  Normal -> Careful [order 1] : [y==3]
  Default -> Normal [order 3] : [y==4]
  data: y input; Buzzer output uint16

== stateflow chart BalanceCar/SetPWM/MotorPinOutput ==
  state PeriodFunction
    en:
    Motor1_A = LOW;
    Motor1_B = LOW;
    Motor2_A = LOW;
    Motor2_B = LOW;
    du:
    Motor1PWM = abs(Motor1PWMTemp);
    Motor2PWM = abs(Motor2PWMTemp);
    SetDirection();
    FallDownDetect();
  state FallDownDetect [function]
    (default) -> (junction 68)
    (junction 68) -> (junction 69) [order 1] : [(Angle > 55) || (Angle < -50)]
    (junction 68) -> (junction 74) [order 2]
    (junction 69) -> (junction 65) : {MotorStop}
    (junction 74) -> (junction 65) [order 1] : [Accel_Z > 18000]
    (junction 74) -> (junction 100) [order 2]
    (junction 65) -> (junction 98)
    (junction 100) -> (junction 98)
  state SetDirection [function]
    (default) -> (junction 9)
    (junction 9) -> (junction 11) [order 1] : [Motor1PWMTemp > NUM0]
    (junction 9) -> (junction 13) [order 2] : {Motor1Backward}
    (junction 11) -> (junction 15) : {Motor1Forward}
    (junction 15) -> (junction 13)
    (junction 13) -> (junction 18)
    (junction 18) -> (junction 19) [order 1] : [Motor2PWMTemp > NUM0]
    (junction 18) -> (junction 29) [order 2] : {Motor2Backward}
    (junction 19) -> (junction 31) : {Motor2Forward}
    (junction 29) -> (junction 31)
  state MotorStop [function]
    (default) -> (junction 62) : {Motor1_A = LOW;
        | Motor1_B = LOW;
        | Motor2_A = LOW;
        | Motor2_B = LOW;
        | Motor1PWM = NUM0;
        | Motor2PWM = NUM0}
  state y=abs(x) [function]
  state Motor1Forward [function]
    (default) -> (junction 48) : {Motor1_A = LOW;
        | Motor1_B = HIGH;}
  state Motor1Backward [function]
    (default) -> (junction 55) : {Motor1_A = HIGH;
        | Motor1_B = LOW;}
  state Motor2Forward [function]
    (default) -> (junction 53) : {Motor2_A = LOW;
        | Motor2_B = HIGH;}
  state Motor2Backward [function]
    (default) -> (junction 57) : {Motor2_A = HIGH;
        | Motor2_B = LOW;}
  (default) -> PeriodFunction
  data: x function_input int16 size=1; y function_output uint16; Motor1PWM output; Motor2PWM output; LOW parameter; Motor1PWMTemp input; Motor2PWMTemp input; Motor1_A output; HIGH parameter; NUM0 parameter; Angle input; Motor1_B output; Motor2_A output; Motor2_B output; Accel_Z input
